simulink model "vhs_fpga_rx_sdram_8k_13xCIC"  (Simulink 7.1)
settings: Solver=FixedStepDiscrete  SolverMode=SingleTasking  StartTime=0.0  StopTime=inf  RelTol=1e-3
undefined symbols (not defined in the file or in its folder): ADC, ADCCIC, ADCClock, BasebandCIC, DAC, Fs, N_frame, N_recv_overlength, VHS
libraries: xbsIndex_r4 x230, vhsadac_common_ob_fpgalib_v1_2_0 x15, misc_tools_fpgalib_v1_0_0 x3, rapid_channel_fpgalib_v1_1_0 x2, misc_tools_dsplib_v1_0_0 x1, sdram_record_playback_fpgalib_v1_0_0 x1, rffe_fpgalib_v1_1_0 x1
(part 3 of 5)

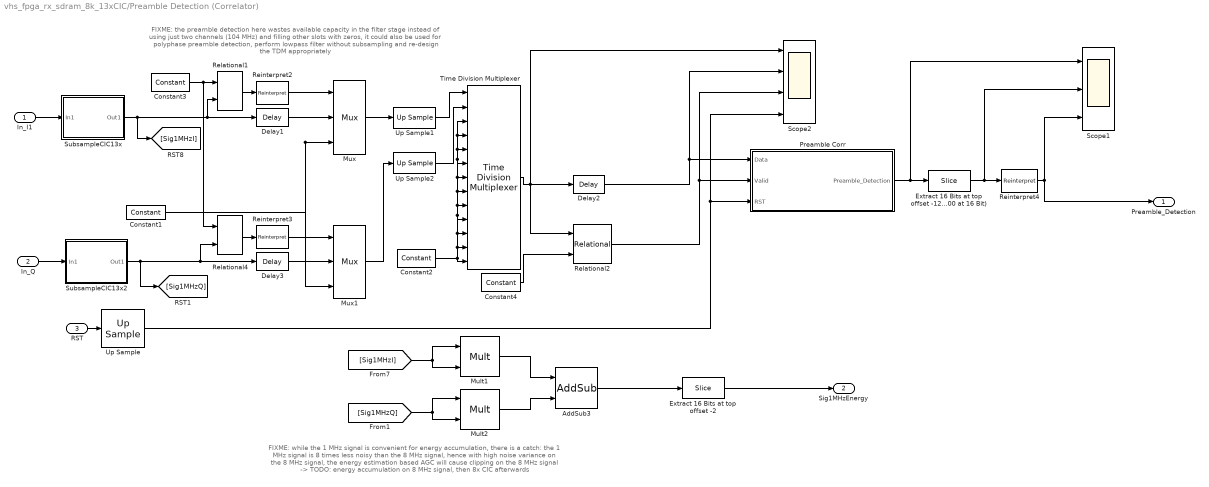
== system vhs_fpga_rx_sdram_8k_13xCIC/Preamble Detection (Correlator) ==
  note: FIXME: while the 1 MHz signal is convenient for energy accumulation, there is a catch:
      | the 1 MHz signal is 8 times less noisy than the 8 MHz signal, hence with high noise variance on the 8 MHz signal, the energy estimation
      | based AGC will cause clipping on the 8 MHz signal -> TODO: energy accumulation on 8 MHz signal, then 8x CIC afterwards
  note: FIXME: the preamble detection here wastes available capacity in the filter stage
      | instead of using just two channels (104 MHz) and filling other slots with zeros, it could also be used for polyphase preamble detection,
      | perform lowpass filter without subsampling and re-design the TDM appropriately
  In_I1 : Inport  OutDataType=sfix(16)  OutScaling=2^0
  In_Q : Inport  Port=2  OutDataType=sfix(16)  OutScaling=2^0
  RST : Inport  Port=3  OutDataType=sfix(16)  OutScaling=2^0
  "   Extract 16 Bits at top offset -12 (room for fully loaded 14 bit input) (offset -16 is barely sufficient for levels of +-4000 at 16 Bit)" : xbsIndex_r4/Slice  nbits=16  boolean_output=off  mode=Upper Bit Location + Width  bit1=-8  base1=MSB of Input  bit0=0  base0=LSB of Input  dbl_ovrd=off  block_type=slice
      settings: infoedit="Extracts a given range of bits from each input sample and presents it at the output.  The output type is ordinarily unsigned with binary point at zero, but can be Boolean when the slice is one bit wide.<P><P>Hardware notes: In hardware this block costs nothing."  block_version=10.1.3
  "   Extract 16 Bits at top offset -2" : xbsIndex_r4/Slice  nbits=16  boolean_output=off  mode=Upper Bit Location + Width  bit1=-2  base1=MSB of Input  bit0=0  base0=LSB of Input  dbl_ovrd=off  block_type=slice
      settings: infoedit="Extracts a given range of bits from each input sample and presents it at the output.  The output type is ordinarily unsigned with binary point at zero, but can be Boolean when the slice is one bit wide.<P><P>Hardware notes: In hardware this block costs nothing."  block_version=10.1.3
  AddSub3 : xbsIndex_r4/AddSub  mode=Addition  use_carryin=off  use_carryout=off  en=off  latency=1  precision=Full  arith_type=Unsigned  n_bits=16  bin_pt=14  quantization=Truncate  overflow=Wrap  dbl_ovrd=off  use_behavioral_HDL=off  pipelined=off  use_rpm=on  hw_selection=Fabric  block_type=addsub
      settings: block_version=10.1.3
  Constant1 : xbsIndex_r4/Constant  arith_type=Signed (2's comp)  const=1  n_bits=16  bin_pt=0  explicit_period=on  period=ADCCIC*BasebandCIC  equ=P=C  opselect=C  inp2=PCIN>>17  opr=+  inp1=P  carry=CIN  dbl_ovrd=off  block_type=constant
  Constant2 : xbsIndex_r4/Constant  arith_type=Signed (2's comp)  const=0  n_bits=16  bin_pt=0  explicit_period=on  period=ADCCIC  equ=P=C  opselect=C  inp2=PCIN>>17  opr=+  inp1=P  carry=CIN  dbl_ovrd=off  block_type=constant
  Constant3 : xbsIndex_r4/Constant  arith_type=Signed (2's comp)  const=0  n_bits=16  bin_pt=13  explicit_period=on  period=ADCCIC*BasebandCIC  equ=P=C  opselect=C  inp2=PCIN>>17  opr=+  inp1=P  carry=CIN  dbl_ovrd=off  block_type=constant
  Constant4 : xbsIndex_r4/Constant  arith_type=Unsigned  const=0  n_bits=2  bin_pt=0  explicit_period=on  period=1  equ=P=C  opselect=C  inp2=PCIN>>17  opr=+  inp1=P  carry=CIN  dbl_ovrd=off  block_type=constant
  Delay1 : xbsIndex_r4/Delay  en=off  latency=1  dbl_ovrd=off  reg_retiming=off  block_type=delay
  Delay2 : xbsIndex_r4/Delay  en=off  latency=1  dbl_ovrd=off  reg_retiming=off  block_type=delay
  Delay3 : xbsIndex_r4/Delay  en=off  latency=1  dbl_ovrd=off  reg_retiming=off  block_type=delay
  Mult1 : xbsIndex_r4/Mult  precision=Full  arith_type="Signed  (2's comp)"  n_bits=16  bin_pt=14  quantization=Truncate  overflow=Wrap  en=off  latency=3  dbl_ovrd=off  use_behavioral_HDL=off  use_embedded=on  opt=Speed  optimum_pipeline=off  pipeline=on  use_rpm=on  placement_style=Triangular  block_type=mult
      settings: infoedit=Hardware notes: To use the internal pipeline stage of the dedicated multiplier you must select 'Pipeline for maximum performance'.  block_version=10.1.3
  Mult2 : xbsIndex_r4/Mult  precision=Full  arith_type="Signed  (2's comp)"  n_bits=16  bin_pt=14  quantization=Truncate  overflow=Wrap  en=off  latency=3  dbl_ovrd=off  use_behavioral_HDL=off  use_embedded=on  opt=Speed  optimum_pipeline=off  pipeline=on  use_rpm=on  placement_style=Triangular  block_type=mult
      settings: infoedit=Hardware notes: To use the internal pipeline stage of the dedicated multiplier you must select 'Pipeline for maximum performance'.  block_version=10.1.3
  Mux : xbsIndex_r4/Mux  inputs=2  en=off  latency=0  precision=Full  arith_type=Unsigned  n_bits=16  bin_pt=14  quantization=Truncate  overflow=Wrap  dbl_ovrd=off  block_type=mux
  Mux1 : xbsIndex_r4/Mux  inputs=2  en=off  latency=0  precision=Full  arith_type=Unsigned  n_bits=16  bin_pt=14  quantization=Truncate  overflow=Wrap  dbl_ovrd=off  block_type=mux
  Preamble Corr : Subsystem
  Reinterpret2 : xbsIndex_r4/Reinterpret  force_arith_type=on  arith_type=Unsigned  force_bin_pt=on  bin_pt=0  block_type=reinterpret
      settings: infoedit="Changes signal type without altering the binary representation.   You can changed the signal between signed and unsigned, and relocate the binary point.<P><P>Hardware notes: In hardware this block costs nothing.<P><P>Example:  Suppose the input is 6 bits wide, signed, with 2 fractional bits, and the output is forced to unsigned with 0 fractional bits.  Then an input of -2.0 (1110.00 in binary 2's complement) becomes an output of 56 (111000 in binary)."  block_version=10.1.3
  Reinterpret3 : xbsIndex_r4/Reinterpret  force_arith_type=on  arith_type=Unsigned  force_bin_pt=on  bin_pt=0  block_type=reinterpret
      settings: infoedit="Changes signal type without altering the binary representation.   You can changed the signal between signed and unsigned, and relocate the binary point.<P><P>Hardware notes: In hardware this block costs nothing.<P><P>Example:  Suppose the input is 6 bits wide, signed, with 2 fractional bits, and the output is forced to unsigned with 0 fractional bits.  Then an input of -2.0 (1110.00 in binary 2's complement) becomes an output of 56 (111000 in binary)."  block_version=10.1.3
  Reinterpret4 : xbsIndex_r4/Reinterpret  force_arith_type=on  arith_type=Unsigned  force_bin_pt=on  bin_pt=0  block_type=reinterpret
      settings: infoedit="Changes signal type without altering the binary representation.   You can changed the signal between signed and unsigned, and relocate the binary point.<P><P>Hardware notes: In hardware this block costs nothing.<P><P>Example:  Suppose the input is 6 bits wide, signed, with 2 fractional bits, and the output is forced to unsigned with 0 fractional bits.  Then an input of -2.0 (1110.00 in binary 2's complement) becomes an output of 56 (111000 in binary)."  block_version=10.1.3
  Relational1 : xbsIndex_r4/Relational  mode=a=b  en=off  latency=1  dbl_ovrd=off  block_type=relational
      settings: block_version=10.1.3
  Relational2 : xbsIndex_r4/Relational  mode=a!=b  en=off  latency=1  dbl_ovrd=off  block_type=relational
      settings: block_version=10.1.3
  Relational4 : xbsIndex_r4/Relational  mode=a=b  en=off  latency=1  dbl_ovrd=off  block_type=relational
      settings: block_version=10.1.3
  Scope1 : Scope  NumInputPorts=3
      settings: YMin=-5~-5~-5  YMax=5~5~5  SaveName=ScopeData4  MaxDataPoints=500000  SampleInput=on
  Scope2 : Scope  NumInputPorts=4
      settings: YMin=-5~-5~-5~-5  YMax=5~5~5~5  SaveName=ScopeData3  MaxDataPoints=500000
  SubsampleCIC13x : Subsystem
  SubsampleCIC13x2 : Subsystem
  Time Division Multiplexer : xbsIndex_r4/Time Division Multiplexer  inputs=13  vin=off  dbl_ovrd=off  explicit_period=off  period=1  block_type=tdm
      settings: infoedit="Multiple inputs are sampled and  presented serially at the output."  block_version=10.1.3
  Up Sample : xbsIndex_r4/Up Sample  sample_ratio=ADCCIC  copy_samples=on  dbl_ovrd=off  block_type=usamp
      settings: infoedit="Up samples input data.  Inserted values  can be zeros or copies of the most recent input sample.<P><P>Hardware notes: No hardware is needed if inserted values are copies of the input sample; otherwise, a mux and single bit flip-flop are used."  block_version=10.1.3
  Up Sample1 : xbsIndex_r4/Up Sample  sample_ratio=BasebandCIC  copy_samples=off  dbl_ovrd=off  block_type=usamp
      settings: infoedit="Up samples input data.  Inserted values  can be zeros or copies of the most recent input sample.<P><P>Hardware notes: No hardware is needed if inserted values are copies of the input sample; otherwise, a mux and single bit flip-flop are used."  block_version=10.1.3
  Up Sample2 : xbsIndex_r4/Up Sample  sample_ratio=BasebandCIC  copy_samples=off  dbl_ovrd=off  block_type=usamp
      settings: infoedit="Up samples input data.  Inserted values  can be zeros or copies of the most recent input sample.<P><P>Hardware notes: No hardware is needed if inserted values are copies of the input sample; otherwise, a mux and single bit flip-flop are used."  block_version=10.1.3
  Preamble_Detection : Outport  OutDataType=sfix(16)  OutScaling=2^0
  Sig1MHzEnergy : Outport  Port=2  OutDataType=sfix(16)  OutScaling=2^0
  wires:
  Preamble Corr/1(Preamble_Detection) -> "   Extract 16 Bits at top offset -12 (room for fully loaded 14 bit input) (offset -16 is barely sufficient for levels of +-4000 at 16 Bit)"/1, Scope1/1
  Time Division Multiplexer/1 -> Delay2/1, Scope2/1, Relational2/1
  In_Q/1 -> SubsampleCIC13x2/1(In1)
  Constant4/1 -> Relational2/2
  RST/1 -> Up Sample/1
  Delay2/1 -> Preamble Corr/1(Data), Scope2/2
  Up Sample/1 -> Preamble Corr/3(RST), Scope2/4
  Relational2/1 -> Preamble Corr/2(Valid), Scope2/3
  Mux/1 -> Up Sample1/1
  Mux1/1 -> Up Sample2/1
  Constant1/1 -> Mux/3, Mux1/3
  Constant3/1 -> Relational1/1, Relational4/1
  Relational1/1 -> Reinterpret2/1
  Relational4/1 -> Reinterpret3/1
  Reinterpret2/1 -> Mux/1
  Reinterpret3/1 -> Mux1/1
  Delay1/1 -> Mux/2
  Delay3/1 -> Mux1/2
  "   Extract 16 Bits at top offset -12 (room for fully loaded 14 bit input) (offset -16 is barely sufficient for levels of +-4000 at 16 Bit)"/1 -> Reinterpret4/1, Scope1/2
  Reinterpret4/1 -> Scope1/3, Preamble_Detection/1
  SubsampleCIC13x/1(Out1) -> Delay1/1, Relational1/2, [Sig1MHzI]
  In_I1/1 -> SubsampleCIC13x/1(In1)
  SubsampleCIC13x2/1(Out1) -> Relational4/2, Delay3/1, [Sig1MHzQ]
  Up Sample1/1 -> Time Division Multiplexer/1
  Up Sample2/1 -> Time Division Multiplexer/2
  [Sig1MHzI] -> Mult1/1, Mult1/2
  [Sig1MHzQ] -> Mult2/2, Mult2/1
  Mult1/1 -> AddSub3/1
  Mult2/1 -> AddSub3/2
  AddSub3/1 -> "   Extract 16 Bits at top offset -2"/1
  "   Extract 16 Bits at top offset -2"/1 -> Sig1MHzEnergy/1
  Constant2/1 -> Time Division Multiplexer/3, Time Division Multiplexer/4, Time Division Multiplexer/5, Time Division Multiplexer/6, Time Division Multiplexer/7, Time Division Multiplexer/8, Time Division Multiplexer/9, Time Division Multiplexer/10, Time Division Multiplexer/11, Time Division Multiplexer/12, Time Division Multiplexer/13

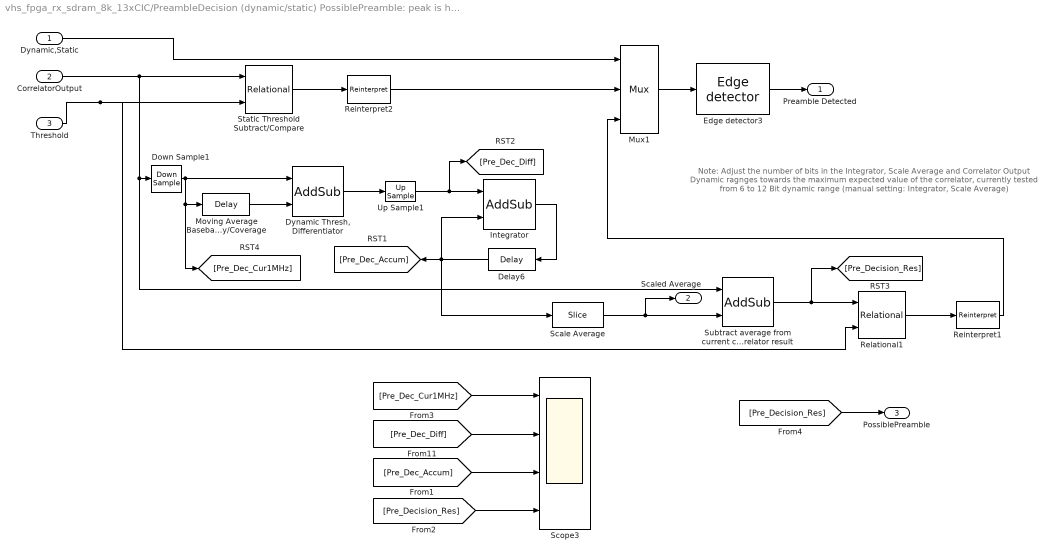
== system vhs_fpga_rx_sdram_8k_13xCIC/PreambleDecision (dynamic/static) PossiblePreamble: peak is higher than ScaledAverage (difference) ==
  note: Note: Adjust the number of bits in the Integrator, Scale Average and Correlator Output Dynamic ragnges
      |  towards the maximum expected value of the correlator, currently tested from 6 to 12 Bit dynamic range
      |  (manual setting: Integrator, Scale Average)
  Dynamic,Static : Inport
  CorrelatorOutput : Inport  Port=2
  Threshold : Inport  Port=3
  Delay6 : xbsIndex_r4/Delay  Orientation=left  en=off  latency=1  dbl_ovrd=off  reg_retiming=off  block_type=delay
  Down Sample1 : xbsIndex_r4/Down Sample  sample_ratio=BasebandCIC  sample_phase="Last Value of Frame  (most efficient)"  en=off  latency=1  dbl_ovrd=off  block_type=dsamp
      settings: block_version=10.1.3
  "Dynamic Thresh, Differentiator" : xbsIndex_r4/AddSub  mode=Subtraction  use_carryin=off  use_carryout=off  en=off  latency=0  precision=Full  arith_type=Unsigned  n_bits=16  bin_pt=14  quantization=Truncate  overflow=Wrap  dbl_ovrd=off  use_behavioral_HDL=off  pipelined=off  use_rpm=on  hw_selection=Fabric  block_type=addsub
      settings: block_version=10.1.3
  Edge detector3 : misc_tools_fpgalib_v1_0_0/Edge detector  Tag=LYR_FPGA_MISC_EDGE_DETECTOR  Description=Lyrtech block  SystemSampleTime=-1  edge_detect=Rising  and_latency=0
  Integrator : xbsIndex_r4/AddSub  mode=Addition  use_carryin=off  use_carryout=off  en=off  latency=0  precision=User Defined  arith_type="Signed  (2's comp)"  n_bits=23  bin_pt=0  quantization=Truncate  overflow=Saturate  dbl_ovrd=off  use_behavioral_HDL=off  pipelined=off  use_rpm=on  hw_selection=Fabric  block_type=addsub
      settings: block_version=10.1.3
  Moving Average Baseband (1MHz) Delay/Coverage : xbsIndex_r4/Delay  en=off  latency=32  dbl_ovrd=off  reg_retiming=off  block_type=delay
  Mux1 : xbsIndex_r4/Mux  inputs=2  en=off  latency=0  precision=Full  arith_type=Unsigned  n_bits=16  bin_pt=14  quantization=Truncate  overflow=Wrap  dbl_ovrd=off  block_type=mux
  Reinterpret1 : xbsIndex_r4/Reinterpret  force_arith_type=on  arith_type=Unsigned  force_bin_pt=on  bin_pt=0  block_type=reinterpret
      settings: infoedit="Changes signal type without altering the binary representation.   You can changed the signal between signed and unsigned, and relocate the binary point.<P><P>Hardware notes: In hardware this block costs nothing.<P><P>Example:  Suppose the input is 6 bits wide, signed, with 2 fractional bits, and the output is forced to unsigned with 0 fractional bits.  Then an input of -2.0 (1110.00 in binary 2's complement) becomes an output of 56 (111000 in binary)."  block_version=10.1.3
  Reinterpret2 : xbsIndex_r4/Reinterpret  force_arith_type=on  arith_type=Unsigned  force_bin_pt=on  bin_pt=0  block_type=reinterpret
      settings: infoedit="Changes signal type without altering the binary representation.   You can changed the signal between signed and unsigned, and relocate the binary point.<P><P>Hardware notes: In hardware this block costs nothing.<P><P>Example:  Suppose the input is 6 bits wide, signed, with 2 fractional bits, and the output is forced to unsigned with 0 fractional bits.  Then an input of -2.0 (1110.00 in binary 2's complement) becomes an output of 56 (111000 in binary)."  block_version=10.1.3
  Relational1 : xbsIndex_r4/Relational  mode=a>=b  en=off  latency=1  dbl_ovrd=off  block_type=relational
      settings: block_version=10.1.3
  Scale Average : xbsIndex_r4/Slice  nbits=16  boolean_output=off  mode=Upper Bit Location + Width  bit1=-6  base1=MSB of Input  bit0=0  base0=LSB of Input  dbl_ovrd=off  block_type=slice
      settings: infoedit="Extracts a given range of bits from each input sample and presents it at the output.  The output type is ordinarily unsigned with binary point at zero, but can be Boolean when the slice is one bit wide.<P><P>Hardware notes: In hardware this block costs nothing."  block_version=10.1.3
  Scope3 : Scope  NumInputPorts=4
      settings: TimeRange=10  YMin=4.75~-9.45~2297~-1155  YMax=5.25~-8.55~2306~-1151  SaveName=ScopeData5  MaxDataPoints=500000
  Static Threshold Subtract/Compare : xbsIndex_r4/Relational  mode=a>=b  en=off  latency=1  dbl_ovrd=off  block_type=relational
      settings: block_version=10.1.3
  Subtract average from current correlator result : xbsIndex_r4/AddSub  mode=Subtraction  use_carryin=off  use_carryout=off  en=off  latency=0  precision=Full  arith_type=Unsigned  n_bits=16  bin_pt=14  quantization=Truncate  overflow=Wrap  dbl_ovrd=off  use_behavioral_HDL=off  pipelined=off  use_rpm=on  hw_selection=Fabric  block_type=addsub
      settings: block_version=10.1.3
  Up Sample1 : xbsIndex_r4/Up Sample  sample_ratio=BasebandCIC  copy_samples=off  dbl_ovrd=off  block_type=usamp
      settings: infoedit="Up samples input data.  Inserted values  can be zeros or copies of the most recent input sample.<P><P>Hardware notes: No hardware is needed if inserted values are copies of the input sample; otherwise, a mux and single bit flip-flop are used."  block_version=10.1.3
  Preamble Detected : Outport
  Scaled Average : Outport  Port=2
  PossiblePreamble : Outport  Port=3
  wires:
  Static Threshold Subtract/Compare/1 -> Reinterpret2/1
  Reinterpret2/1 -> Mux1/2
  Moving Average Baseband (1MHz) Delay/Coverage/1 -> "Dynamic Thresh, Differentiator"/2
  "Dynamic Thresh, Differentiator"/1 -> Up Sample1/1
  Integrator/1 -> Delay6/1
  Delay6/1 -> Integrator/2, [Pre_Dec_Accum], Scale Average/1
  Scale Average/1 -> Subtract average from current correlator result/2, Scaled Average/1
  Reinterpret1/1 -> Mux1/3
  Relational1/1 -> Reinterpret1/1
  Down Sample1/1 -> "Dynamic Thresh, Differentiator"/1, Moving Average Baseband (1MHz) Delay/Coverage/1, [Pre_Dec_Cur1MHz]
  CorrelatorOutput/1 -> Static Threshold Subtract/Compare/1, Down Sample1/1, Subtract average from current correlator result/1
  Dynamic,Static/1 -> Mux1/1
  Mux1/1 -> Edge detector3/1
  Edge detector3/1 -> Preamble Detected/1
  Threshold/1 -> Static Threshold Subtract/Compare/2, Relational1/2
  [Pre_Dec_Diff] -> Scope3/2
  [Pre_Dec_Accum] -> Scope3/3
  Subtract average from current correlator result/1 -> Relational1/1, [Pre_Decision_Res]
  [Pre_Decision_Res] -> Scope3/4
  [Pre_Dec_Cur1MHz] -> Scope3/1
  Up Sample1/1 -> Integrator/1, [Pre_Dec_Diff]
  [Pre_Decision_Res] -> PossiblePreamble/1

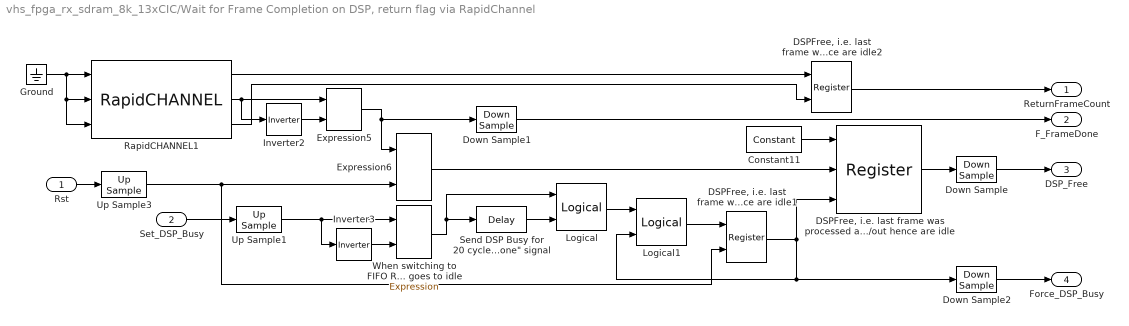
== system vhs_fpga_rx_sdram_8k_13xCIC/Wait for Frame Completion on DSP, return flag via RapidChannel ==
  Rst : Inport
  Set_DSP_Busy : Inport  Port=2
  "  When switching to FIFO READ (RC write), clear DSP Free Bit, note: rising edge detector in principle not necessary, as the DSP can only be \"done\" after the whole frame is transmitted, i.e. after the read state is done and the state machine goes to idle" : xbsIndex_r4/Expression  expression=a & b  align_bp=on  en=off  latency=0  precision=Full  arith_type=Unsigned  n_bits=16  bin_pt=0  dbl_ovrd=off  block_type=expr
      settings: block_version=10.1.3
  Constant11 : xbsIndex_r4/Constant  arith_type=Boolean  const=0  n_bits=1  bin_pt=0  explicit_period=on  period=1  equ=P=C  opselect=C  inp2=PCIN>>17  opr=+  inp1=P  carry=CIN  dbl_ovrd=off  block_type=constant
  "DSPFree, i.e. last frame was processed and FastBus in/out hence are idle" : xbsIndex_r4/Register  init=1  rst=on  en=on  dbl_ovrd=off  block_type=register
  "DSPFree, i.e. last frame was processed and FastBus in/out hence are idle1" : xbsIndex_r4/Register  init=0  rst=on  en=off  dbl_ovrd=off  block_type=register
  "DSPFree, i.e. last frame was processed and FastBus in/out hence are idle2" : xbsIndex_r4/Register  init=0  rst=off  en=on  dbl_ovrd=off  block_type=register
  Down Sample : xbsIndex_r4/Down Sample  sample_ratio=ADCCIC  sample_phase="Last Value of Frame  (most efficient)"  en=off  latency=1  dbl_ovrd=off  block_type=dsamp
      settings: block_version=10.1.3
  Down Sample1 : xbsIndex_r4/Down Sample  sample_ratio=ADCCIC  sample_phase="Last Value of Frame  (most efficient)"  en=off  latency=1  dbl_ovrd=off  block_type=dsamp
      settings: block_version=10.1.3
  Down Sample2 : xbsIndex_r4/Down Sample  sample_ratio=ADCCIC  sample_phase="Last Value of Frame  (most efficient)"  en=off  latency=1  dbl_ovrd=off  block_type=dsamp
      settings: block_version=10.1.3
  Expression5 : xbsIndex_r4/Expression  expression=a & b  align_bp=on  en=off  latency=0  precision=Full  arith_type=Unsigned  n_bits=16  bin_pt=0  dbl_ovrd=off  block_type=expr
      settings: block_version=10.1.3
  Expression6 : xbsIndex_r4/Expression  expression=a | b  align_bp=on  en=off  latency=0  precision=Full  arith_type=Unsigned  n_bits=16  bin_pt=0  dbl_ovrd=off  block_type=expr
      settings: block_version=10.1.3
  Ground : Ground
  Inverter2 : xbsIndex_r4/Inverter  en=off  latency=1  dbl_ovrd=off  block_type=inv
  Inverter3 : xbsIndex_r4/Inverter  en=off  latency=1  dbl_ovrd=off  block_type=inv
  Logical : xbsIndex_r4/Logical  logical_function=XOR  inputs=2  en=off  latency=0  precision=Full  arith_type=Unsigned  n_bits=16  bin_pt=0  align_bp=on  dbl_ovrd=off  block_type=logical
  Logical1 : xbsIndex_r4/Logical  logical_function=XOR  inputs=2  en=off  latency=0  precision=Full  arith_type=Unsigned  n_bits=16  bin_pt=0  align_bp=on  dbl_ovrd=off  block_type=logical
  RapidCHANNEL1 : rapid_channel_fpgalib_v1_1_0/RapidCHANNEL  Tag=LYR_FPGA_IO_RAPIDCHANNEL  Description=Lyrtech block  SystemSampleTime=-1  board_type=VHS-ADC/DAC  interface_quad=LYRIO  interface_drc=LYRIO  interface_dual=LYRIO  direction=RX  output_arithmetic_type=Unsigned  output_width=32  binpt=0  sample_period=1  provide_control=off  provide_pio=off  pio1_direction=Input
  "Send DSP Busy for 20 cycles to avoid wrong Free state with slow SMQ \"frame_done\" signal" : xbsIndex_r4/Delay  en=off  latency=20  dbl_ovrd=off  reg_retiming=off  block_type=delay
  Up Sample1 : xbsIndex_r4/Up Sample  sample_ratio=ADCCIC  copy_samples=on  dbl_ovrd=off  block_type=usamp
      settings: infoedit="Up samples input data.  Inserted values  can be zeros or copies of the most recent input sample.<P><P>Hardware notes: No hardware is needed if inserted values are copies of the input sample; otherwise, a mux and single bit flip-flop are used."  block_version=10.1.3
  Up Sample3 : xbsIndex_r4/Up Sample  sample_ratio=ADCCIC  copy_samples=on  dbl_ovrd=off  block_type=usamp
      settings: infoedit="Up samples input data.  Inserted values  can be zeros or copies of the most recent input sample.<P><P>Hardware notes: No hardware is needed if inserted values are copies of the input sample; otherwise, a mux and single bit flip-flop are used."  block_version=10.1.3
  ReturnFrameCount : Outport
  F_FrameDone : Outport  Port=2
  DSP_Free : Outport  Port=3
  Force_DSP_Busy : Outport  Port=4
  wires:
  RapidCHANNEL1/3 -> "DSPFree, i.e. last frame was processed and FastBus in/out hence are idle2"/2
  RapidCHANNEL1/1 -> "DSPFree, i.e. last frame was processed and FastBus in/out hence are idle2"/1
  "DSPFree, i.e. last frame was processed and FastBus in/out hence are idle1"/1 -> "DSPFree, i.e. last frame was processed and FastBus in/out hence are idle"/3, Logical1/2, Down Sample2/1
  Logical1/1 -> "DSPFree, i.e. last frame was processed and FastBus in/out hence are idle1"/1
  "  When switching to FIFO READ (RC write), clear DSP Free Bit, note: rising edge detector in principle not necessary, as the DSP can only be \"done\" after the whole frame is transmitted, i.e. after the read state is done and the state machine goes to idle"/1 -> "Send DSP Busy for 20 cycles to avoid wrong Free state with slow SMQ \"frame_done\" signal"/1, Logical/1
  Logical/1 -> Logical1/1
  "Send DSP Busy for 20 cycles to avoid wrong Free state with slow SMQ \"frame_done\" signal"/1 -> Logical/2
  Up Sample1/1 -> "  When switching to FIFO READ (RC write), clear DSP Free Bit, note: rising edge detector in principle not necessary, as the DSP can only be \"done\" after the whole frame is transmitted, i.e. after the read state is done and the state machine goes to idle"/1, Inverter3/1
  Inverter3/1 -> "  When switching to FIFO READ (RC write), clear DSP Free Bit, note: rising edge detector in principle not necessary, as the DSP can only be \"done\" after the whole frame is transmitted, i.e. after the read state is done and the state machine goes to idle"/2
  "DSPFree, i.e. last frame was processed and FastBus in/out hence are idle"/1 -> Down Sample/1
  Rst/1 -> Up Sample3/1
  Expression5/1 -> Expression6/1, Down Sample1/1
  Expression6/1 -> "DSPFree, i.e. last frame was processed and FastBus in/out hence are idle"/2
  RapidCHANNEL1/2 -> Inverter2/1, Expression5/1
  Inverter2/1 -> Expression5/2
  Constant11/1 -> "DSPFree, i.e. last frame was processed and FastBus in/out hence are idle"/1
  Ground/1 -> RapidCHANNEL1/2, RapidCHANNEL1/3, RapidCHANNEL1/1
  "DSPFree, i.e. last frame was processed and FastBus in/out hence are idle2"/1 -> ReturnFrameCount/1
  Down Sample1/1 -> F_FrameDone/1
  Down Sample/1 -> DSP_Free/1
  Set_DSP_Busy/1 -> Up Sample1/1
  Down Sample2/1 -> Force_DSP_Busy/1
  Up Sample3/1 -> "DSPFree, i.e. last frame was processed and FastBus in/out hence are idle1"/2, Expression6/2

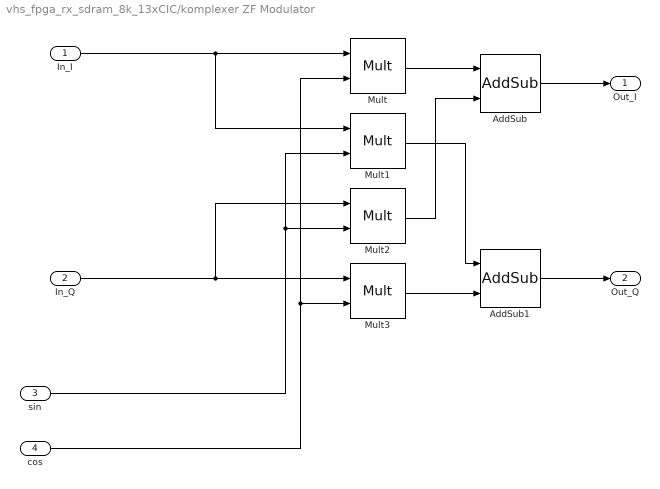
== system vhs_fpga_rx_sdram_8k_13xCIC/komplexer ZF Modulator ==
  In_I : Inport  OutDataType=sfix(16)  OutScaling=2^0
  In_Q : Inport  Port=2  OutDataType=sfix(16)  OutScaling=2^0
  sin : Inport  Port=3  OutDataType=sfix(16)  OutScaling=2^0
  cos : Inport  Port=4  OutDataType=sfix(16)  OutScaling=2^0
  AddSub : xbsIndex_r4/AddSub  mode=Subtraction  use_carryin=off  use_carryout=off  en=off  latency=0  precision=User Defined  arith_type="Signed  (2's comp)"  n_bits=14  bin_pt=0  quantization=Truncate  overflow=Wrap  dbl_ovrd=off  use_behavioral_HDL=off  pipelined=off  use_rpm=on  hw_selection=Fabric  block_type=addsub
      settings: xl_area=[7 0 0 14 0 0 0]  block_version=9.2.00
  AddSub1 : xbsIndex_r4/AddSub  mode=Addition  use_carryin=off  use_carryout=off  en=off  latency=0  precision=User Defined  arith_type="Signed  (2's comp)"  n_bits=14  bin_pt=0  quantization=Truncate  overflow=Wrap  dbl_ovrd=off  use_behavioral_HDL=off  pipelined=off  use_rpm=on  hw_selection=Fabric  block_type=addsub
      settings: xl_area=[7 0 0 14 0 0 0]  block_version=9.2.00
  Mult{,1..3} (4 alike) : xbsIndex_r4/Mult  precision=User Defined  arith_type="Signed  (2's comp)"  n_bits=14  bin_pt=0  quantization=Truncate  overflow=Wrap  en=off  latency=3  dbl_ovrd=off  use_behavioral_HDL=off  use_embedded=on  opt=Speed  optimum_pipeline=off  pipeline=on  use_rpm=on  placement_style=Triangular  block_type=mult
      settings: infoedit=Hardware notes: To use the internal pipeline stage of the dedicated multiplier you must select 'Pipeline for maximum performance'.  xl_area=[17 34 0 14 0 1 0]  block_version=9.2.00
  Out_I : Outport  OutDataType=sfix(16)  OutScaling=2^0
  Out_Q : Outport  Port=2  OutDataType=sfix(16)  OutScaling=2^0
  wires:
  Mult3/1 -> AddSub1/2
  Mult/1 -> AddSub/1
  AddSub/1 -> Out_I/1
  AddSub1/1 -> Out_Q/1
  In_I/1 -> Mult/1, Mult1/1
  In_Q/1 -> Mult3/1, Mult2/1
  Mult2/1 -> AddSub/2
  Mult1/1 -> AddSub1/1
  sin/1 -> Mult2/2, Mult1/2
  cos/1 -> Mult3/2, Mult/2

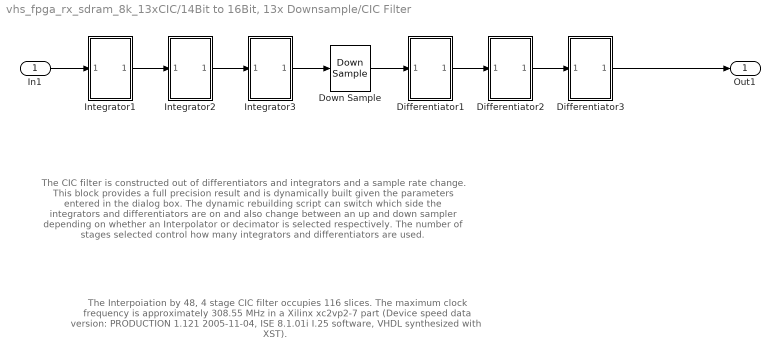
== system vhs_fpga_rx_sdram_8k_13xCIC/14Bit to 16Bit, 13x Downsample/CIC Filter ==
  note: The CIC filter is constructed out of differentiators and integrators and
      | a sample rate change. This block provides a full precision result and is
      | dynamically built given the parameters entered in the dialog box. The
      | dynamic rebuilding script can switch which side the integrators and
      | differentiators are on and also change between an up and down sampler
      | depending on whether an Interpolator or decimator is selected respectively.
      | The number of stages selected control how many integrators and
      | differentiators are used.
  note: The Interpoiation by 48, 4 stage CIC filter occupies 116 slices.
      | The maximum clock frequency is approximately
      | 308.55 MHz in a Xilinx xc2vp2-7 part (Device speed data version:
      | PRODUCTION 1.121 2005-11-04, ISE 8.1.01i I.25 software, VHDL
      | synthesized with XST).
  In1 : Inport  OutDataType=sfix(16)  OutScaling=2^0
  Differentiator1 : Subsystem  mask(Differentiator Stage){m=m, output_bitwidth=ceil(stages*log2(rate_change*m) + input_bitwidth), output_binpt=input_binpt}
      mask prompts: m "Differential Delay"; output_bitwidth "Output Bit Width"; output_binpt "Output Binary Point"
      mask help: Multi-Channel Differentiator
      mask init:
      | set_param(gcb, 'LinkStatus', 'none');
  Differentiator2 : Subsystem  mask(Differentiator Stage){m=m, output_bitwidth=ceil(stages*log2(rate_change*m) + input_bitwidth), output_binpt=input_binpt}
      mask prompts: m "Differential Delay"; output_bitwidth "Output Bit Width"; output_binpt "Output Binary Point"
      mask help: Multi-Channel Differentiator
      mask init:
      | set_param(gcb, 'LinkStatus', 'none');
  Differentiator3 : Subsystem  mask(Differentiator Stage){m=m, output_bitwidth=ceil(stages*log2(rate_change*m) + input_bitwidth), output_binpt=input_binpt}
      mask prompts: m "Differential Delay"; output_bitwidth "Output Bit Width"; output_binpt "Output Binary Point"
      mask help: Multi-Channel Differentiator
      mask init:
      | set_param(gcb, 'LinkStatus', 'none');
  Down Sample : xbsIndex_r4/Down Sample  sample_ratio=rate_change  sample_phase=First Value of Frame  en=off  latency=1  dbl_ovrd=off  block_type=dsamp
      settings: block_version=9.2.00
  Integrator1 : Subsystem  mask(Integrator Stage){output_bitwidth=ceil(stages*log2(rate_change*m) + input_bitwidth)}
      mask prompts: output_bitwidth "Output Bit Width"
      mask help: Multi Channel Integrator
      mask init:
      | set_param(gcb, 'LinkStatus', 'none');
      settings: CopyFcn=set_param(gcb, 'LinkStatus', 'none');
  Integrator2 : Subsystem  mask(Integrator Stage){output_bitwidth=ceil(stages*log2(rate_change*m) + input_bitwidth)}
      mask prompts: output_bitwidth "Output Bit Width"
      mask help: Multi Channel Integrator
      mask init:
      | set_param(gcb, 'LinkStatus', 'none');
      settings: CopyFcn=set_param(gcb, 'LinkStatus', 'none');
  Integrator3 : Subsystem  mask(Integrator Stage){output_bitwidth=ceil(stages*log2(rate_change*m) + input_bitwidth)}
      mask prompts: output_bitwidth "Output Bit Width"
      mask help: Multi Channel Integrator
      mask init:
      | set_param(gcb, 'LinkStatus', 'none');
      settings: CopyFcn=set_param(gcb, 'LinkStatus', 'none');
  Out1 : Outport  OutDataType=sfix(16)  OutScaling=2^0
  wires:
  In1/1 -> Integrator1/1(In1)
  Down Sample/1 -> Differentiator1/1(In1)
  Integrator1/1(Out1) -> Integrator2/1(In1)
  Differentiator1/1(Out1) -> Differentiator2/1(In1)
  Integrator2/1(Out1) -> Integrator3/1(In1)
  Differentiator2/1(Out1) -> Differentiator3/1(In1)
  Integrator3/1(Out1) -> Down Sample/1
  Differentiator3/1(Out1) -> Out1/1

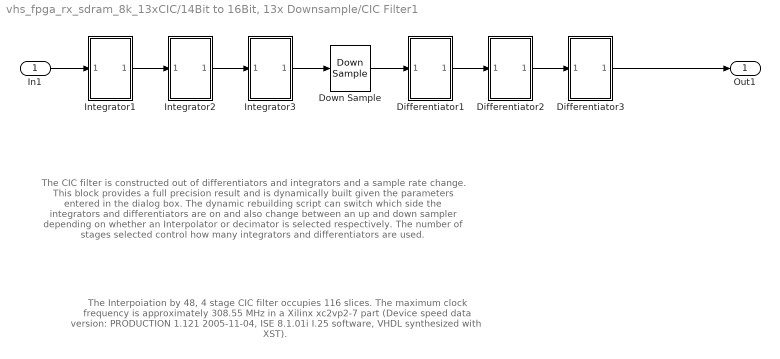
== system vhs_fpga_rx_sdram_8k_13xCIC/14Bit to 16Bit, 13x Downsample/CIC Filter1 ==
  note: The CIC filter is constructed out of differentiators and integrators and
      | a sample rate change. This block provides a full precision result and is
      | dynamically built given the parameters entered in the dialog box. The
      | dynamic rebuilding script can switch which side the integrators and
      | differentiators are on and also change between an up and down sampler
      | depending on whether an Interpolator or decimator is selected respectively.
      | The number of stages selected control how many integrators and
      | differentiators are used.
  note: The Interpoiation by 48, 4 stage CIC filter occupies 116 slices.
      | The maximum clock frequency is approximately
      | 308.55 MHz in a Xilinx xc2vp2-7 part (Device speed data version:
      | PRODUCTION 1.121 2005-11-04, ISE 8.1.01i I.25 software, VHDL
      | synthesized with XST).
  In1 : Inport  OutDataType=sfix(16)  OutScaling=2^0
  Differentiator1 : Subsystem  mask(Differentiator Stage){m=m, output_bitwidth=ceil(stages*log2(rate_change*m) + input_bitwidth), output_binpt=input_binpt}
      mask prompts: m "Differential Delay"; output_bitwidth "Output Bit Width"; output_binpt "Output Binary Point"
      mask help: Multi-Channel Differentiator
      mask init:
      | set_param(gcb, 'LinkStatus', 'none');
  Differentiator2 : Subsystem  mask(Differentiator Stage){m=m, output_bitwidth=ceil(stages*log2(rate_change*m) + input_bitwidth), output_binpt=input_binpt}
      mask prompts: m "Differential Delay"; output_bitwidth "Output Bit Width"; output_binpt "Output Binary Point"
      mask help: Multi-Channel Differentiator
      mask init:
      | set_param(gcb, 'LinkStatus', 'none');
  Differentiator3 : Subsystem  mask(Differentiator Stage){m=m, output_bitwidth=ceil(stages*log2(rate_change*m) + input_bitwidth), output_binpt=input_binpt}
      mask prompts: m "Differential Delay"; output_bitwidth "Output Bit Width"; output_binpt "Output Binary Point"
      mask help: Multi-Channel Differentiator
      mask init:
      | set_param(gcb, 'LinkStatus', 'none');
  Down Sample : xbsIndex_r4/Down Sample  sample_ratio=rate_change  sample_phase=First Value of Frame  en=off  latency=1  dbl_ovrd=off  block_type=dsamp
      settings: block_version=9.2.00
  Integrator1 : Subsystem  mask(Integrator Stage){output_bitwidth=ceil(stages*log2(rate_change*m) + input_bitwidth)}
      mask prompts: output_bitwidth "Output Bit Width"
      mask help: Multi Channel Integrator
      mask init:
      | set_param(gcb, 'LinkStatus', 'none');
      settings: CopyFcn=set_param(gcb, 'LinkStatus', 'none');
  Integrator2 : Subsystem  mask(Integrator Stage){output_bitwidth=ceil(stages*log2(rate_change*m) + input_bitwidth)}
      mask prompts: output_bitwidth "Output Bit Width"
      mask help: Multi Channel Integrator
      mask init:
      | set_param(gcb, 'LinkStatus', 'none');
      settings: CopyFcn=set_param(gcb, 'LinkStatus', 'none');
  Integrator3 : Subsystem  mask(Integrator Stage){output_bitwidth=ceil(stages*log2(rate_change*m) + input_bitwidth)}
      mask prompts: output_bitwidth "Output Bit Width"
      mask help: Multi Channel Integrator
      mask init:
      | set_param(gcb, 'LinkStatus', 'none');
      settings: CopyFcn=set_param(gcb, 'LinkStatus', 'none');
  Out1 : Outport  OutDataType=sfix(16)  OutScaling=2^0
  wires:
  In1/1 -> Integrator1/1(In1)
  Down Sample/1 -> Differentiator1/1(In1)
  Integrator1/1(Out1) -> Integrator2/1(In1)
  Differentiator1/1(Out1) -> Differentiator2/1(In1)
  Integrator2/1(Out1) -> Integrator3/1(In1)
  Differentiator2/1(Out1) -> Differentiator3/1(In1)
  Integrator3/1(Out1) -> Down Sample/1
  Differentiator3/1(Out1) -> Out1/1

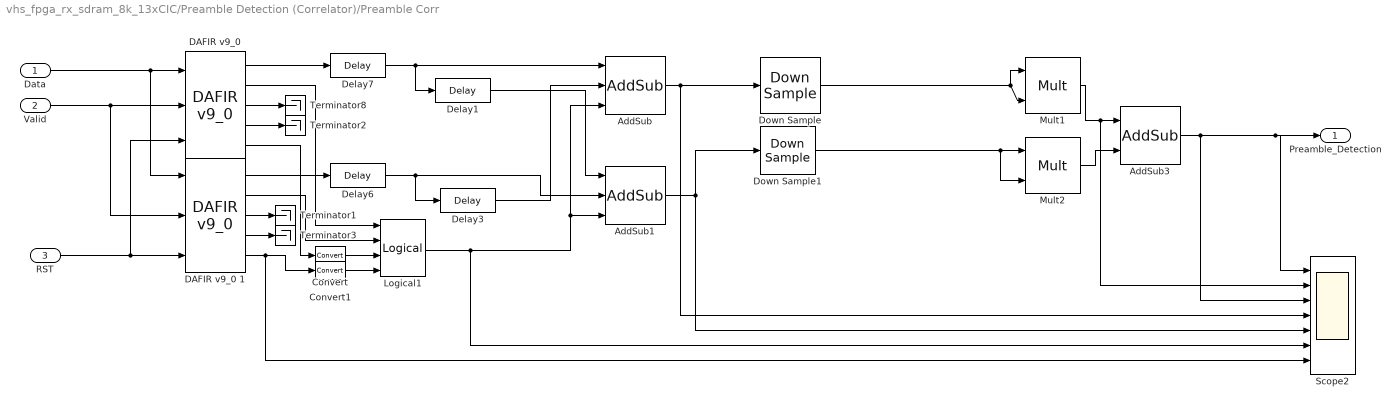
== system vhs_fpga_rx_sdram_8k_13xCIC/Preamble Detection (Correlator)/Preamble Corr ==
  Data : Inport  OutDataType=sfix(16)  OutScaling=2^0
  Valid : Inport  Port=2  OutDataType=sfix(16)  OutScaling=2^0
  RST : Inport  Port=3  OutDataType=sfix(16)  OutScaling=2^0
  AddSub : xbsIndex_r4/AddSub  mode=Addition  use_carryin=off  use_carryout=off  en=on  latency=1  precision=Full  arith_type=Unsigned  n_bits=16  bin_pt=14  quantization=Truncate  overflow=Wrap  dbl_ovrd=off  use_behavioral_HDL=off  pipelined=off  use_rpm=on  hw_selection=Fabric  block_type=addsub
      settings: block_version=10.1.3
  AddSub1 : xbsIndex_r4/AddSub  mode=Subtraction  use_carryin=off  use_carryout=off  en=on  latency=1  precision=Full  arith_type=Unsigned  n_bits=16  bin_pt=14  quantization=Truncate  overflow=Wrap  dbl_ovrd=off  use_behavioral_HDL=off  pipelined=off  use_rpm=on  hw_selection=Fabric  block_type=addsub
      settings: block_version=10.1.3
  AddSub3 : xbsIndex_r4/AddSub  mode=Addition  use_carryin=off  use_carryout=off  en=off  latency=1  precision=Full  arith_type=Unsigned  n_bits=16  bin_pt=14  quantization=Truncate  overflow=Wrap  dbl_ovrd=off  use_behavioral_HDL=off  pipelined=off  use_rpm=on  hw_selection=Fabric  block_type=addsub
      settings: block_version=10.1.3
  Convert : xbsIndex_r4/Convert  arith_type=Boolean  n_bits=16  bin_pt=14  quantization=Truncate  overflow=Wrap  latency=0  dbl_ovrd=off  pipeline=off  block_type=convert
      settings: block_version=10.1.3
  Convert1 : xbsIndex_r4/Convert  arith_type=Boolean  n_bits=16  bin_pt=14  quantization=Truncate  overflow=Wrap  latency=0  dbl_ovrd=off  pipeline=off  block_type=convert
      settings: block_version=10.1.3
  "DAFIR v9_0 " : xbsIndex_r4/DAFIR v9_0   coef=2^8 * real( conj([(longPreamble_time(end:-1:1))]) )  structure=Inferred from Coefficients  coef_n_bits=10  coef_bin_pt=0  over_sample=1  reload=off  valids=on  rst=on  latency=12  num_channels=2  serial_input=on  polyphase_behavior="Single Rate:  sample in - sample out"  dbl_ovrd=off  explicit_period=off  period=1  use_isim=0  block_type=fir
      settings: infoedit="Hardware notes: Implemented using distributed arithmetic (DA).  The hardware over sampling rate determines the degree of parallelism.  A rate of one produces a fully parallel DA filter.  A rate of n (resp., n+1) for an n-bit input signal produces a fully serial implementation for a non-symmetric (resp., symmetric) impulse response.  Intermediate values produce implementations with intermediate levels of parallelism."  block_version=10.1.3
  DAFIR v9_0 1 : xbsIndex_r4/DAFIR v9_0   coef=2^8 * imag( conj([(longPreamble_time(end:-1:1))]) )  structure=Inferred from Coefficients  coef_n_bits=10  coef_bin_pt=0  over_sample=1  reload=off  valids=on  rst=on  latency=12  num_channels=2  serial_input=on  polyphase_behavior="Single Rate:  sample in - sample out"  dbl_ovrd=off  explicit_period=off  period=1  use_isim=0  block_type=fir
      settings: infoedit="Hardware notes: Implemented using distributed arithmetic (DA).  The hardware over sampling rate determines the degree of parallelism.  A rate of one produces a fully parallel DA filter.  A rate of n (resp., n+1) for an n-bit input signal produces a fully serial implementation for a non-symmetric (resp., symmetric) impulse response.  Intermediate values produce implementations with intermediate levels of parallelism."  block_version=10.1.3
  Delay{1,3,6..7} (4 alike) : xbsIndex_r4/Delay  en=off  latency=1  dbl_ovrd=off  reg_retiming=off  block_type=delay
  Down Sample : xbsIndex_r4/Down Sample  sample_ratio=ADCCIC  sample_phase="Last Value of Frame  (most efficient)"  en=off  latency=1  dbl_ovrd=off  block_type=dsamp
      settings: block_version=10.1.3
  Down Sample1 : xbsIndex_r4/Down Sample  sample_ratio=ADCCIC  sample_phase="Last Value of Frame  (most efficient)"  en=off  latency=1  dbl_ovrd=off  block_type=dsamp
      settings: block_version=10.1.3
  Logical1 : xbsIndex_r4/Logical  logical_function=AND  inputs=4  en=off  latency=1  precision=Full  arith_type=Unsigned  n_bits=16  bin_pt=0  align_bp=on  dbl_ovrd=off  block_type=logical
  Mult1 : xbsIndex_r4/Mult  precision=Full  arith_type="Signed  (2's comp)"  n_bits=16  bin_pt=14  quantization=Truncate  overflow=Wrap  en=off  latency=3  dbl_ovrd=off  use_behavioral_HDL=off  use_embedded=on  opt=Speed  optimum_pipeline=off  pipeline=on  use_rpm=on  placement_style=Triangular  block_type=mult
      settings: infoedit=Hardware notes: To use the internal pipeline stage of the dedicated multiplier you must select 'Pipeline for maximum performance'.  block_version=10.1.3
  Mult2 : xbsIndex_r4/Mult  precision=Full  arith_type="Signed  (2's comp)"  n_bits=16  bin_pt=14  quantization=Truncate  overflow=Wrap  en=off  latency=3  dbl_ovrd=off  use_behavioral_HDL=off  use_embedded=on  opt=Speed  optimum_pipeline=off  pipeline=on  use_rpm=on  placement_style=Triangular  block_type=mult
      settings: infoedit=Hardware notes: To use the internal pipeline stage of the dedicated multiplier you must select 'Pipeline for maximum performance'.  block_version=10.1.3
  Scope2 : Scope  NumInputPorts=7
      settings: YMin=-5~-5~-5~-5~-5~-5~-5  YMax=5~5~5~5~5~5~5  MaxDataPoints=500000
  Terminator{1..3,8} (4 alike) : Terminator
  Preamble_Detection : Outport  OutDataType=sfix(16)  OutScaling=2^0
  wires:
  "DAFIR v9_0 "/2 -> Logical1/1
  DAFIR v9_0 1/2 -> Logical1/2
  "DAFIR v9_0 "/1 -> Delay7/1
  DAFIR v9_0 1/1 -> Delay6/1
  Delay7/1 -> Delay1/1, AddSub/1
  Delay6/1 -> Delay3/1, AddSub1/2
  Delay3/1 -> AddSub/2
  Logical1/1 -> AddSub1/3, AddSub/3, Scope2/6
  "DAFIR v9_0 "/5 -> Convert/1
  DAFIR v9_0 1/5 -> Convert1/1, Scope2/7
  Convert/1 -> Logical1/3
  Convert1/1 -> Logical1/4
  AddSub1/1 -> Scope2/5, Down Sample1/1
  Valid/1 -> DAFIR v9_0 1/2, "DAFIR v9_0 "/2
  Data/1 -> "DAFIR v9_0 "/1, DAFIR v9_0 1/1
  RST/1 -> "DAFIR v9_0 "/3, DAFIR v9_0 1/3
  Delay1/1 -> AddSub1/1
  AddSub/1 -> Scope2/4, Down Sample/1
  AddSub3/1 -> Scope2/3, Preamble_Detection/1, Scope2/1
  Mult1/1 -> AddSub3/1, Scope2/2
  Mult2/1 -> AddSub3/2
  Down Sample/1 -> Mult1/1, Mult1/2
  Down Sample1/1 -> Mult2/1, Mult2/2
  "DAFIR v9_0 "/3 -> Terminator8/1
  "DAFIR v9_0 "/4 -> Terminator2/1
  DAFIR v9_0 1/3 -> Terminator1/1
  DAFIR v9_0 1/4 -> Terminator3/1
